simulink model "DSMC_Plus_DeadZone"  (R2019b)
settings: Solver=VariableStepAuto  StartTime=0.0  StopTime=100  RelTol=1e-3
settings Model: Creator=Asus  LastModifiedBy=Asus

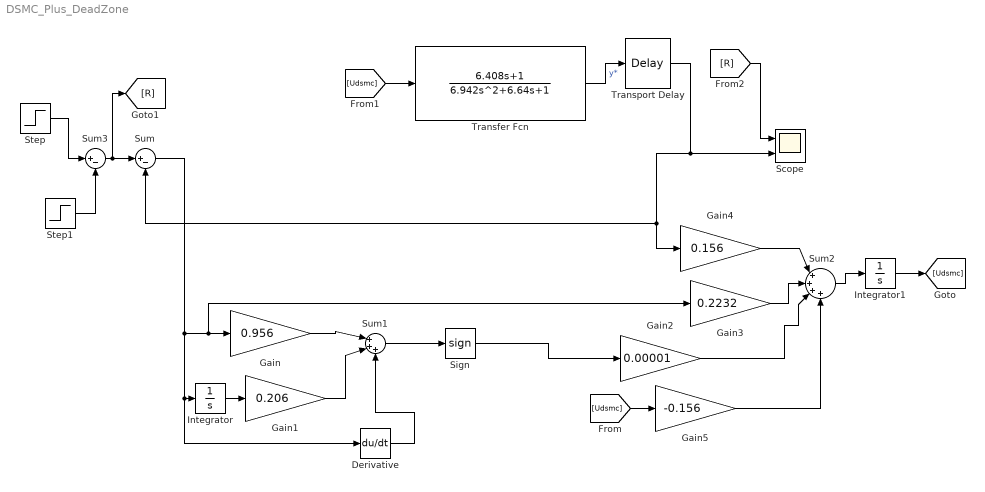
== system DSMC_Plus_DeadZone ==
  Derivative : Derivative
  Gain : Gain  Gain=0.956
  Gain1 : Gain  Gain=0.206
  Gain2 : Gain  Gain=0.00001
  Gain3 : Gain  Gain=0.2232
  Gain4 : Gain  Gain=0.156
  Gain5 : Gain  Gain=-0.156
  Integrator : Integrator
  Integrator1 : Integrator
  Scope : Scope  NumInputPorts=2
  Sign : Signum
  Step : Step  Time=5  SampleTime=0
  Step1 : Step  Time=60  After=0.5  SampleTime=0
  Sum : Sum  Inputs=|+-
  Sum1 : Sum  Inputs=|+++
  Sum2 : Sum  Inputs=|++++
  Sum3 : Sum  Inputs=|+-
  Transfer Fcn : TransferFcn  Numerator=[6.408 1]  Denominator=[6.942 6.64 1]
  Transport Delay : TransportDelay  DelayTime=6
  wires:
  Step/1 -> Sum3/1
  Sum3/1 -> [R], Sum/1
  Sum/1 -> Gain3/1, Gain/1, Derivative/1, Integrator/1
  Sign/1 -> Gain2/1
  Gain1/1 -> Sum1/2
  Derivative/1 -> Sum1/3
  Integrator/1 -> Gain1/1
  Gain5/1 -> Sum2/4
  Gain/1 -> Sum1/1
  Sum1/1 -> Sign/1
  [R] -> Scope/1
  Integrator1/1 -> [Udsmc]
  [Udsmc] -> Gain5/1
  Step1/1 -> Sum3/2
  [Udsmc] -> Transfer Fcn/1
  Sum2/1 -> Integrator1/1
  Gain4/1 -> Sum2/1
  Gain2/1 -> Sum2/3
  Gain3/1 -> Sum2/2
  Transport Delay/1 -> Scope/2, Sum/2, Gain4/1
  Transfer Fcn/1 -> Transport Delay/1  "y*"
